simulink model "main_09_simulink"  (R2022a)
settings: Solver=VariableStepAuto  StartTime=0.0  StopTime=50  RelTol=1e-3
values from neighbouring files (symbols this model uses):
  u1 = 60.9532    [main_09.m]
  u2 = 25.0223    [main_09.m]
  u3 = 39.2577    [main_09.m]
  u4 = 44.1767    [main_09.m]
settings Model: Creator=Eshmith  LastModifiedBy=Eshmith

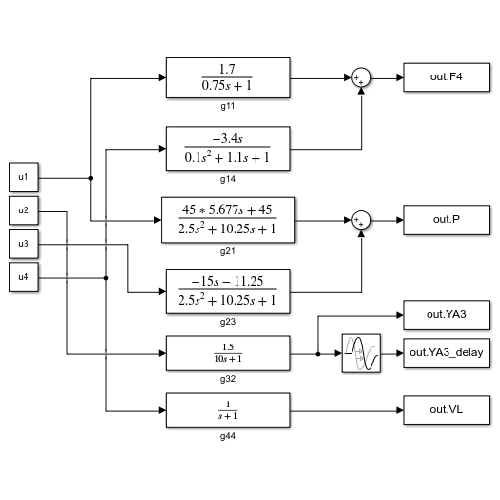
[thumbnail: Simulink's stored preview of the top-level diagram]
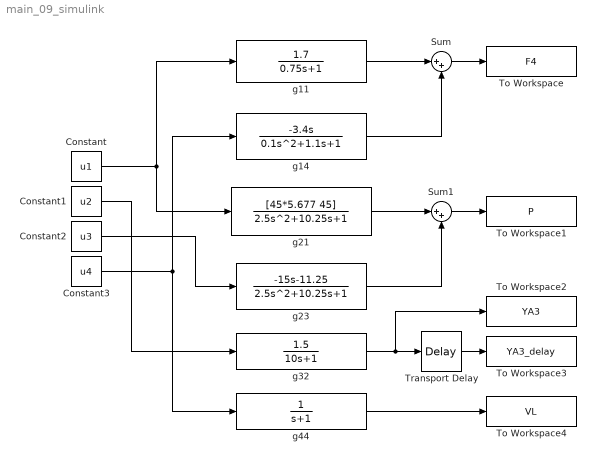
== system main_09_simulink ==
  Constant : Constant  Value=u1
  Constant1 : Constant  Value=u2
  Constant2 : Constant  Value=u3
  Constant3 : Constant  Value=u4
  Sum : Sum  Inputs=|++
  Sum1 : Sum  Inputs=|++
  To Workspace : ToWorkspace  VariableName=F4  SaveFormat=Timeseries  SampleTime=-1
  To Workspace1 : ToWorkspace  VariableName=P  SaveFormat=Timeseries  SampleTime=-1
  To Workspace2 : ToWorkspace  VariableName=YA3  SaveFormat=Timeseries  SampleTime=-1
  To Workspace3 : ToWorkspace  VariableName=YA3_delay  SaveFormat=Timeseries  SampleTime=-1
  To Workspace4 : ToWorkspace  VariableName=VL  SaveFormat=Timeseries  SampleTime=-1
  Transport Delay : TransportDelay  DelayTime=0.1
  g11 : TransferFcn  Numerator=[1.7]  Denominator=[0.75 1]
  g14 : TransferFcn  Numerator=[-3.4 0]  Denominator=[0.1 1.1 1]
  g21 : TransferFcn  Numerator=[45*5.677 45]  Denominator=[2.5 10.25 1]
  g23 : TransferFcn  Numerator=[-15 -11.25]  Denominator=[2.5 10.25 1]
  g32 : TransferFcn  Numerator=[1.5]  Denominator=[10 1]
  g44 : TransferFcn  Denominator=[1 1]
  wires:
  Constant/1 -> g11/1, g21/1
  g32/1 -> Transport Delay/1, To Workspace2/1
  Sum1/1 -> To Workspace1/1
  g44/1 -> To Workspace4/1
  Constant1/1 -> g32/1
  Sum/1 -> To Workspace/1
  g21/1 -> Sum1/1
  Constant2/1 -> g23/1
  Transport Delay/1 -> To Workspace3/1
  Constant3/1 -> g14/1, g44/1
  g14/1 -> Sum/2
  g23/1 -> Sum1/2
  g11/1 -> Sum/1
